simulink model "DIMR_ordinary"  (R2024b)
settings: Solver=daessc  StartTime=0.0  StopTime=60  RelTol=1e-3
values from neighbouring files (symbols this model uses):
  d_m0 = d_mn    (= 0)    [DIMR_main.m]
  d_m_cmd = 0.12787808985686    (= 0.127878089857)    [DIMR_main.m]
  dis_cmd = 0    [DIMR_main.m]
  jrk_cmd = 0.15    [DIMR_main.m]
  phi_cmd = 0*pi/180    (= 0)    [DIMR_main.m]
  ta = (vel_cmd-jrk_cmd*tt^2)/acc_cmd    (= 3.66666666667)    [DIMR_main.m]
  taz = z_vel_cmd/z_acc_cmd    (= 1.6)    [DIMR_main.m]
  tc = (x_cmd-2*(1/2*acc_cmd*ta^2+1/2*jrk_cmd*tt^2*ta+tt*vel_cmd))/vel_cmd    (= 10.6666666667)    [DIMR_main.m]
  tcz = (z_cmd-z_acc_cmd*taz^2)/z_vel_cmd    [DIMR_main.m]
  tcz2 = (z_cmd2-z_acc_cmd*taz^2)/z_vel_cmd    (= 0.9)    [DIMR_main.m]
  theta_f0 = -theta_p0    (= -0.024)    [DIMR_main.m]
  theta_f_cmd = 0.037940459    [DIMR_main.m]
  theta_p0 = theta_pn    (= 0.024)    [DIMR_main.m]
  theta_p_cmd = -0.037940459    [DIMR_main.m]
  ts = 15    [DIMR_main.m]
  ts2 = te+5    (= 39.3333333333)    [DIMR_main.m]
  tsz = 10    [DIMR_main.m]
  tsz2 = ts2    (= 39.3333333333)    [DIMR_main.m]
  tt = acc_cmd/jrk_cmd    (= 0.333333333333)    [DIMR_main.m]
  x_cmd = 3    [DIMR_main.m]
  z_0 = R_wo+L_bmy+L_my/2    [DIMR_main.m]
  z_acc_cmd = 0.05    [DIMR_main.m]
  z_cmd = 0.9-z_0    [DIMR_main.m]
  z_cmd2 = 0.9-0.7    (= 0.2)    [DIMR_main.m]
undefined symbols (not defined in the file or in its folder): Ac, Dc, DiscIntNeverNeededParam, dspblkCoreblockFVToolHelper, g, g_ext, g_fork, g_lift, g_reac, g_spado, g_yaw, gcbh, K_fd, K_fp, K_md, K_mp, K_pd, K_pp, K_wd, K_wi, K_wp, K_yd, K_yp, Kc, L_bg, L_bmx, L_bmy, L_bmz, L_bsx, L_bsy, L_bsz, L_by, L_ex, L_ey, L_ez, L_fg, L_fh, L_fx, L_fy, L_fz, L_lx, L_ly, L_lz, L_mg, L_mx, L_my, L_mz, L_wt, M_b, M_f, M_m, M_n11, M_n21, M_n22, M_n33, M_n44, Mc, N_f, N_w, omega_c ... (+10)
libraries: simulink x56, sm_lib x54, nesl_utility x12, slctrl_autotuning x1, slpidlib x1
(part 2 of 6)

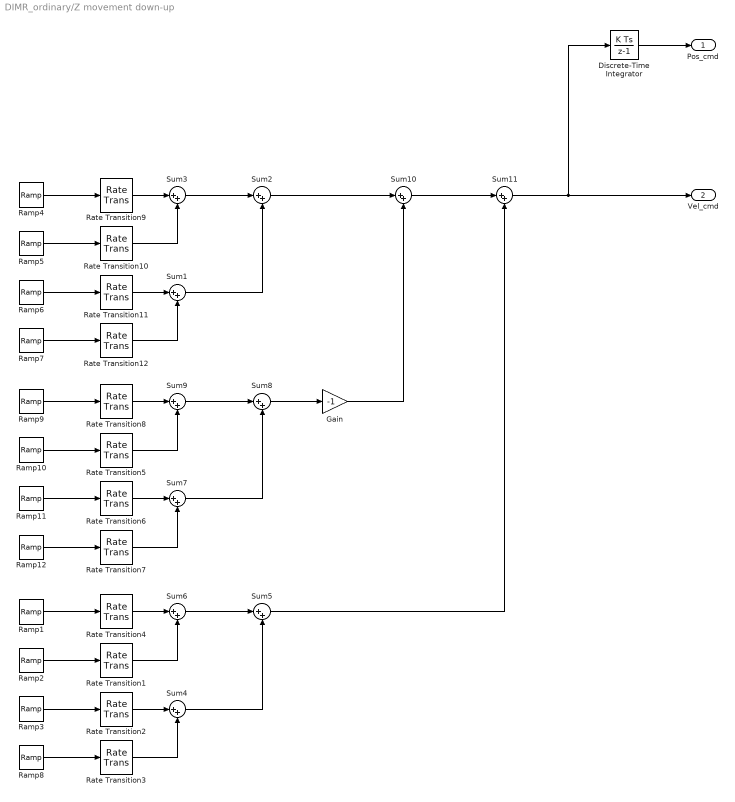
== system DIMR_ordinary/Z movement down-up ==
  Discrete-Time Integrator : DiscreteIntegrator  InitialCondition=z_0  SampleTime=T_control  ICPrevOutput=DiscIntNeverNeededParam  ICPrevScaledInput=DiscIntNeverNeededParam
  Gain : Gain  Gain=-1
  Ramp1 : simulink/Sources/Ramp  slope=z_acc_cmd  start=24  InitialOutput=0
  Ramp10 : simulink/Sources/Ramp  slope=-z_acc_cmd  start=17+taz  InitialOutput=0
  Ramp11 : simulink/Sources/Ramp  slope=-z_acc_cmd  start=17+taz+tcz  InitialOutput=0
  Ramp12 : simulink/Sources/Ramp  slope=z_acc_cmd  start=17+tcz+2*taz  InitialOutput=0
  Ramp2 : simulink/Sources/Ramp  slope=-z_acc_cmd  start=24+taz  InitialOutput=0
  Ramp3 : simulink/Sources/Ramp  slope=-z_acc_cmd  start=24+taz+tcz  InitialOutput=0
  Ramp4 : simulink/Sources/Ramp  slope=z_acc_cmd  start=tsz  InitialOutput=0
  Ramp5 : simulink/Sources/Ramp  slope=-z_acc_cmd  start=tsz+taz  InitialOutput=0
  Ramp6 : simulink/Sources/Ramp  slope=-z_acc_cmd  start=tsz+taz+tcz  InitialOutput=0
  Ramp7 : simulink/Sources/Ramp  slope=z_acc_cmd  start=tsz+tcz+2*taz  InitialOutput=0
  Ramp8 : simulink/Sources/Ramp  slope=z_acc_cmd  start=24+tcz+2*taz  InitialOutput=0
  Ramp9 : simulink/Sources/Ramp  slope=z_acc_cmd  start=17  InitialOutput=0
  Rate Transition{1..12} (12 alike) : RateTransition  OutPortSampleTime=T_control
  Sum{1..11} (11 alike) : Sum  Inputs=|++
  Pos_cmd : Outport
  Vel_cmd : Outport  Port=2
  wires:
  Discrete-Time Integrator/1 -> Pos_cmd/1
  Ramp7/1 -> Rate Transition12/1
  Ramp5/1 -> Rate Transition10/1
  Sum3/1 -> Sum2/1
  Sum1/1 -> Sum2/2
  Rate Transition10/1 -> Sum3/2
  Ramp6/1 -> Rate Transition11/1
  Ramp4/1 -> Rate Transition9/1
  Rate Transition12/1 -> Sum1/2
  Rate Transition11/1 -> Sum1/1
  Rate Transition9/1 -> Sum3/1
  Rate Transition4/1 -> Sum6/1
  Rate Transition2/1 -> Sum4/1
  Rate Transition3/1 -> Sum4/2
  Ramp1/1 -> Rate Transition4/1
  Ramp3/1 -> Rate Transition2/1
  Rate Transition1/1 -> Sum6/2
  Sum4/1 -> Sum5/2
  Sum6/1 -> Sum5/1
  Ramp2/1 -> Rate Transition1/1
  Ramp8/1 -> Rate Transition3/1
  Ramp12/1 -> Rate Transition7/1
  Ramp10/1 -> Rate Transition5/1
  Sum9/1 -> Sum8/1
  Sum7/1 -> Sum8/2
  Rate Transition5/1 -> Sum9/2
  Ramp11/1 -> Rate Transition6/1
  Ramp9/1 -> Rate Transition8/1
  Rate Transition7/1 -> Sum7/2
  Rate Transition6/1 -> Sum7/1
  Rate Transition8/1 -> Sum9/1
  Sum8/1 -> Gain/1
  Sum2/1 -> Sum10/1
  Gain/1 -> Sum10/2
  Sum5/1 -> Sum11/2
  Sum10/1 -> Sum11/1
  Sum11/1 -> Discrete-Time Integrator/1, Vel_cmd/1

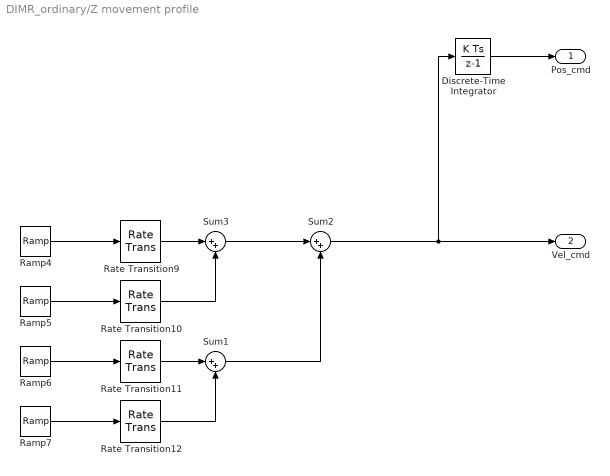
== system DIMR_ordinary/Z movement profile ==
  Discrete-Time Integrator : DiscreteIntegrator  InitialCondition=z_0  SampleTime=T_control  ICPrevOutput=DiscIntNeverNeededParam  ICPrevScaledInput=DiscIntNeverNeededParam
  Ramp4 : simulink/Sources/Ramp  slope=z_acc_cmd  start=tsz  InitialOutput=0
  Ramp5 : simulink/Sources/Ramp  slope=-z_acc_cmd  start=tsz+taz  InitialOutput=0
  Ramp6 : simulink/Sources/Ramp  slope=-z_acc_cmd  start=tsz+taz+tcz  InitialOutput=0
  Ramp7 : simulink/Sources/Ramp  slope=z_acc_cmd  start=tsz+tcz+2*taz  InitialOutput=0
  Rate Transition{9..12} (4 alike) : RateTransition  OutPortSampleTime=T_control
  Sum1 : Sum  Inputs=|++
  Sum2 : Sum  Inputs=|++
  Sum3 : Sum  Inputs=|++
  Pos_cmd : Outport
  Vel_cmd : Outport  Port=2
  wires:
  Rate Transition9/1 -> Sum3/1
  Rate Transition11/1 -> Sum1/1
  Rate Transition12/1 -> Sum1/2
  Ramp4/1 -> Rate Transition9/1
  Ramp6/1 -> Rate Transition11/1
  Sum2/1 -> Discrete-Time Integrator/1, Vel_cmd/1
  Rate Transition10/1 -> Sum3/2
  Sum1/1 -> Sum2/2
  Sum3/1 -> Sum2/1
  Ramp5/1 -> Rate Transition10/1
  Ramp7/1 -> Rate Transition12/1
  Discrete-Time Integrator/1 -> Pos_cmd/1

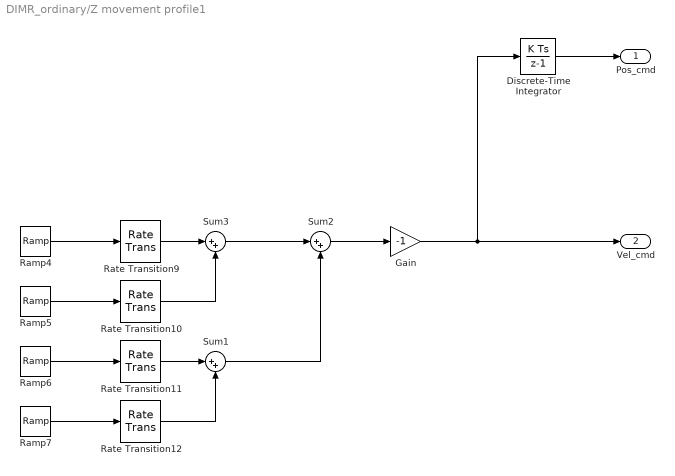
== system DIMR_ordinary/Z movement profile1 ==
  Discrete-Time Integrator : DiscreteIntegrator  InitialCondition=z_0+z_cmd  SampleTime=T_control  ICPrevOutput=DiscIntNeverNeededParam  ICPrevScaledInput=DiscIntNeverNeededParam
  Gain : Gain  Gain=-1
  Ramp4 : simulink/Sources/Ramp  slope=z_acc_cmd  start=tsz2  InitialOutput=0
  Ramp5 : simulink/Sources/Ramp  slope=-z_acc_cmd  start=tsz2+taz  InitialOutput=0
  Ramp6 : simulink/Sources/Ramp  slope=-z_acc_cmd  start=tsz2+taz+tcz2  InitialOutput=0
  Ramp7 : simulink/Sources/Ramp  slope=z_acc_cmd  start=tsz2+tcz2+2*taz  InitialOutput=0
  Rate Transition{9..12} (4 alike) : RateTransition  OutPortSampleTime=T_control
  Sum1 : Sum  Inputs=|++
  Sum2 : Sum  Inputs=|++
  Sum3 : Sum  Inputs=|++
  Pos_cmd : Outport
  Vel_cmd : Outport  Port=2
  wires:
  Discrete-Time Integrator/1 -> Pos_cmd/1
  Gain/1 -> Discrete-Time Integrator/1, Vel_cmd/1
  Ramp4/1 -> Rate Transition9/1
  Ramp7/1 -> Rate Transition12/1
  Rate Transition12/1 -> Sum1/2
  Rate Transition9/1 -> Sum3/1
  Ramp6/1 -> Rate Transition11/1
  Sum3/1 -> Sum2/1
  Sum1/1 -> Sum2/2
  Rate Transition10/1 -> Sum3/2
  Rate Transition11/1 -> Sum1/1
  Ramp5/1 -> Rate Transition10/1
  Sum2/1 -> Gain/1
